simulink model "MainAssembly1"  (R2023a)
settings: Solver=VariableStepAuto  StartTime=0.0  StopTime=0.25  RelTol=1e-3
model workspace: external: MATLAB File C:\Users\danen\Desktop\MQPTest\MainAssembly1_DataFile1.m (data not in the file)
values from neighbouring files (symbols this model uses):
  Ts = 1e-06    [MainAssembly1_DataFile1.m]
undefined symbols (not defined in the file or in its folder): DiscIntNeverNeededParam, smiData, X, Y, Z
libraries: sm_lib x165, fl_lib x20, nesl_utility x10, fl_ps_legacy_lib x8, spsUniversalBridgeLib x8, spsCurrentMeasurementLib x8, spsDCVoltageSourceLib x4, spsStepperMotorLib x4, ee_lib x2, simulink x1, sps_lib x1
(part 1 of 4)
settings Model: Creator=danen  LastModifiedBy=danen

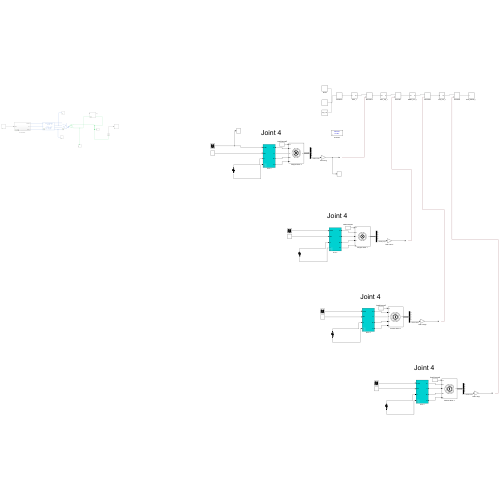
[thumbnail: Simulink's stored preview of the top-level diagram]
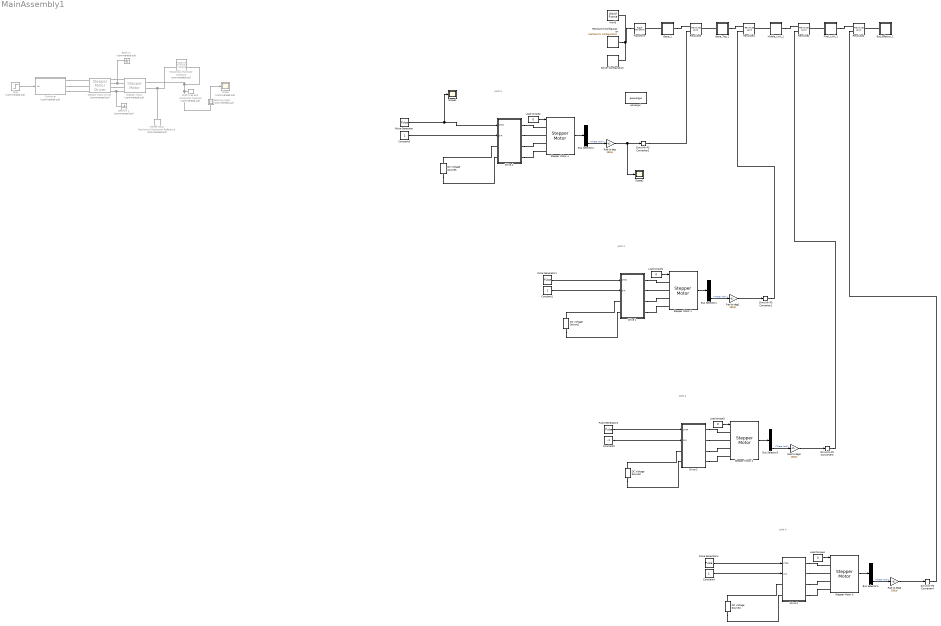
== system MainAssembly1 ==
  note: Joint 4
  note: Joint 4
  note: Joint 4
  note: Joint 4
  Base_1 : Subsystem
  Base_Top_1 : Subsystem
  Bus Selector{1..4} (4 alike) : BusSelector  OutputSignals=Vph (V),Iph (A),Te (N*m),w (rad/s),Theta (rad)
  Constant1 : Constant
  Constant2 : Constant  Value=-1
  Constant3 : Constant
  Constant4 : Constant
  Controller : Subsystem  Commented=on  Variant=on  VariantControlMode=label  LabelModeActiveChoice=Position
      settings: AttributesFormatString=%<BlockChoice>
  DC Voltage Source{1..4} (4 alike) : spsDCVoltageSourceLib/DC Voltage Source  Amplitude=5  Measurements=None
  Drive 1 : Subsystem  mask{Iref=2, step=500, Ts=Ts}
      mask prompts: Iref "Phase current (A)"; step "Stepping rate (step/s)"; Ts "Sampling time (s)"
      mask init:
      | Nstep=round(1/step/Ts);
  Drive 2 : Subsystem  mask{Iref=2, step=500, Ts=Ts}
      mask prompts: Iref "Phase current (A)"; step "Stepping rate (step/s)"; Ts "Sampling time (s)"
      mask init:
      | Nstep=round(1/step/Ts);
  Drive 3 : Subsystem  mask{Iref=2, step=500, Ts=Ts}
      mask prompts: Iref "Phase current (A)"; step "Stepping rate (step/s)"; Ts "Sampling time (s)"
      mask init:
      | Nstep=round(1/step/Ts);
  Drive 4 : Subsystem  mask{Iref=2, step=500, Ts=Ts}
      mask prompts: Iref "Phase current (A)"; step "Stepping rate (step/s)"; Ts "Sampling time (s)"
      mask init:
      | Nstep=round(1/step/Ts);
  ERef A+ : fl_lib/Electrical/Electrical Elements/Electrical Reference  Commented=on
  ERef A+1 : fl_lib/Electrical/Electrical Elements/Electrical Reference  Commented=on
  End_Effector_1 : Subsystem
  Final_Link_1 : Subsystem
  Load torque{1..4} (4 alike) : Constant  Value=0
  MRRef Motor : fl_lib/Mechanical/Rotational Elements/Mechanical Rotational Reference  Commented=on
  MechanismConfiguration : sm_lib/Utilities/Mechanism Configuration  UniformGravity=Constant  GravityVector=[0 -9.80665 0]  GravityVectorUnits=m/s^2  LinearizationDelta=0.001  JointModeTransitionNonlinearIterations=2
  Middle_Link_1 : Subsystem
  Pulse Generator : DiscretePulseGenerator  PulseType=Time based  Period=0.2  PulseWidth=0.5
  Pulse Generator1 : DiscretePulseGenerator  PulseType=Time based  Period=0.1  PulseWidth=0.1
  Pulse Generator2 : DiscretePulseGenerator  PulseType=Time based  Period=0.1  PulseWidth=0.1
  Pulse Generator4 : DiscretePulseGenerator  PulseType=Time based  Period=0.1  PulseWidth=0.1
  Rad to deg{,1..3} (4 alike) : Gain  Gain=180/pi
  Revolute1 : sm_lib/Joints/Revolute Joint  JointMode=Normal  SenseConstraintForce=off  SenseConstraintForceX=off  SenseConstraintForceY=off  SenseConstraintForceZ=off  SenseConstraintTorque=off  SenseConstraintTorqueX=off  SenseConstraintTorqueY=off  SenseConstraintTorqueZ=off  SenseTotalForce=off  SenseTotalForceX=off  SenseTotalForceY=off  SenseTotalForceZ=off  SenseTotalTorque=off  SenseTotalTorqueX=off  SenseTotalTorqueY=off  SenseTotalTorqueZ=off  CompositeWrenchDir=FollowerOnBase  CompositeWrenchFrame=BaseFrame  EquilibriumPosition=0  EquilibriumPositionUnits=deg  SpringStiffness=0  SpringStiffnessUnits=N*m/deg  DampingCoefficient=0  DampingCoefficientUnits=N*m/(deg/s)  TorqueActuationMode=ComputedTorque  MotionActuationMode=InputMotion  SensePosition=off  SenseVelocity=off  SenseAcceleration=off  SenseTorqueForce=off  SenseLowerLimitTorqueForce=off  SenseUpperLimitTorqueForce=off  LowerLimitSpecify=off  LowerLimitBound=-90  LowerLimitBoundUnits=deg  LowerLimitStiffness=1e4  LowerLimitStiffnessUnits=N*m/deg  LowerLimitDamping=10  LowerLimitDampingUnits=N*m/(deg/s)  LowerLimitTransitionRegionWidth=0.1  LowerLimitTransitionRegionWidthUnits=deg  UpperLimitSpecify=off  UpperLimitBound=90  UpperLimitBoundUnits=deg  UpperLimitStiffness=1e4  UpperLimitStiffnessUnits=N*m/deg  UpperLimitDamping=10  UpperLimitDampingUnits=N*m/(deg/s)  UpperLimitTransitionRegionWidth=0.1  UpperLimitTransitionRegionWidthUnits=deg  PositionTargetSpecify=on  PositionTargetPriority=Low  PositionTargetValue=smiData.RevoluteJoint(3).Rz.Pos  PositionTargetValueUnits=deg  VelocityTargetSpecify=off  VelocityTargetPriority=High  VelocityTargetValue=0  VelocityTargetValueUnits=deg/s
  Revolute2 : sm_lib/Joints/Revolute Joint  JointMode=Normal  SenseConstraintForce=off  SenseConstraintForceX=off  SenseConstraintForceY=off  SenseConstraintForceZ=off  SenseConstraintTorque=off  SenseConstraintTorqueX=off  SenseConstraintTorqueY=off  SenseConstraintTorqueZ=off  SenseTotalForce=off  SenseTotalForceX=off  SenseTotalForceY=off  SenseTotalForceZ=off  SenseTotalTorque=off  SenseTotalTorqueX=off  SenseTotalTorqueY=off  SenseTotalTorqueZ=off  CompositeWrenchDir=FollowerOnBase  CompositeWrenchFrame=BaseFrame  EquilibriumPosition=0  EquilibriumPositionUnits=deg  SpringStiffness=0  SpringStiffnessUnits=N*m/deg  DampingCoefficient=0  DampingCoefficientUnits=N*m/(deg/s)  TorqueActuationMode=ComputedTorque  MotionActuationMode=InputMotion  SensePosition=off  SenseVelocity=off  SenseAcceleration=off  SenseTorqueForce=off  SenseLowerLimitTorqueForce=off  SenseUpperLimitTorqueForce=off  LowerLimitSpecify=off  LowerLimitBound=-90  LowerLimitBoundUnits=deg  LowerLimitStiffness=1e4  LowerLimitStiffnessUnits=N*m/deg  LowerLimitDamping=10  LowerLimitDampingUnits=N*m/(deg/s)  LowerLimitTransitionRegionWidth=0.1  LowerLimitTransitionRegionWidthUnits=deg  UpperLimitSpecify=off  UpperLimitBound=90  UpperLimitBoundUnits=deg  UpperLimitStiffness=1e4  UpperLimitStiffnessUnits=N*m/deg  UpperLimitDamping=10  UpperLimitDampingUnits=N*m/(deg/s)  UpperLimitTransitionRegionWidth=0.1  UpperLimitTransitionRegionWidthUnits=deg  PositionTargetSpecify=on  PositionTargetPriority=Low  PositionTargetValue=smiData.RevoluteJoint(1).Rz.Pos  PositionTargetValueUnits=deg  VelocityTargetSpecify=off  VelocityTargetPriority=High  VelocityTargetValue=0  VelocityTargetValueUnits=deg/s
  Revolute3 : sm_lib/Joints/Revolute Joint  JointMode=Normal  SenseConstraintForce=off  SenseConstraintForceX=off  SenseConstraintForceY=off  SenseConstraintForceZ=off  SenseConstraintTorque=off  SenseConstraintTorqueX=off  SenseConstraintTorqueY=off  SenseConstraintTorqueZ=off  SenseTotalForce=off  SenseTotalForceX=off  SenseTotalForceY=off  SenseTotalForceZ=off  SenseTotalTorque=off  SenseTotalTorqueX=off  SenseTotalTorqueY=off  SenseTotalTorqueZ=off  CompositeWrenchDir=FollowerOnBase  CompositeWrenchFrame=BaseFrame  EquilibriumPosition=0  EquilibriumPositionUnits=deg  SpringStiffness=0  SpringStiffnessUnits=N*m/deg  DampingCoefficient=0  DampingCoefficientUnits=N*m/(deg/s)  TorqueActuationMode=ComputedTorque  MotionActuationMode=InputMotion  SensePosition=off  SenseVelocity=off  SenseAcceleration=off  SenseTorqueForce=off  SenseLowerLimitTorqueForce=off  SenseUpperLimitTorqueForce=off  LowerLimitSpecify=off  LowerLimitBound=-90  LowerLimitBoundUnits=deg  LowerLimitStiffness=1e4  LowerLimitStiffnessUnits=N*m/deg  LowerLimitDamping=10  LowerLimitDampingUnits=N*m/(deg/s)  LowerLimitTransitionRegionWidth=0.1  LowerLimitTransitionRegionWidthUnits=deg  UpperLimitSpecify=off  UpperLimitBound=90  UpperLimitBoundUnits=deg  UpperLimitStiffness=1e4  UpperLimitStiffnessUnits=N*m/deg  UpperLimitDamping=10  UpperLimitDampingUnits=N*m/(deg/s)  UpperLimitTransitionRegionWidth=0.1  UpperLimitTransitionRegionWidthUnits=deg  PositionTargetSpecify=on  PositionTargetPriority=Low  PositionTargetValue=smiData.RevoluteJoint(4).Rz.Pos  PositionTargetValueUnits=deg  VelocityTargetSpecify=off  VelocityTargetPriority=High  VelocityTargetValue=0  VelocityTargetValueUnits=deg/s
  Revolute4 : sm_lib/Joints/Revolute Joint  JointMode=Normal  SenseConstraintForce=off  SenseConstraintForceX=off  SenseConstraintForceY=off  SenseConstraintForceZ=off  SenseConstraintTorque=off  SenseConstraintTorqueX=off  SenseConstraintTorqueY=off  SenseConstraintTorqueZ=off  SenseTotalForce=off  SenseTotalForceX=off  SenseTotalForceY=off  SenseTotalForceZ=off  SenseTotalTorque=off  SenseTotalTorqueX=off  SenseTotalTorqueY=off  SenseTotalTorqueZ=off  CompositeWrenchDir=FollowerOnBase  CompositeWrenchFrame=BaseFrame  EquilibriumPosition=0  EquilibriumPositionUnits=deg  SpringStiffness=0  SpringStiffnessUnits=N*m/deg  DampingCoefficient=0  DampingCoefficientUnits=N*m/(deg/s)  TorqueActuationMode=ComputedTorque  MotionActuationMode=InputMotion  SensePosition=off  SenseVelocity=off  SenseAcceleration=off  SenseTorqueForce=off  SenseLowerLimitTorqueForce=off  SenseUpperLimitTorqueForce=off  LowerLimitSpecify=off  LowerLimitBound=-90  LowerLimitBoundUnits=deg  LowerLimitStiffness=1e4  LowerLimitStiffnessUnits=N*m/deg  LowerLimitDamping=10  LowerLimitDampingUnits=N*m/(deg/s)  LowerLimitTransitionRegionWidth=0.1  LowerLimitTransitionRegionWidthUnits=deg  UpperLimitSpecify=off  UpperLimitBound=90  UpperLimitBoundUnits=deg  UpperLimitStiffness=1e4  UpperLimitStiffnessUnits=N*m/deg  UpperLimitDamping=10  UpperLimitDampingUnits=N*m/(deg/s)  UpperLimitTransitionRegionWidth=0.1  UpperLimitTransitionRegionWidthUnits=deg  PositionTargetSpecify=on  PositionTargetPriority=Low  PositionTargetValue=smiData.RevoluteJoint(2).Rz.Pos  PositionTargetValueUnits=deg  VelocityTargetSpecify=off  VelocityTargetPriority=High  VelocityTargetValue=0  VelocityTargetValueUnits=deg/s
  Rotational Multibody Interface : fl_lib/Mechanical/Multibody Interfaces/Rotational Multibody Interface  Commented=on
  Scope : Scope  Commented=on
  Scope1 : Scope
  Scope2 : Scope
  Sensing Angle : Subsystem  Commented=on
      mask Display: disp('a')
  Shaft Free End : fl_lib/Mechanical/Rotational Elements/Rotational Free End  Commented=on  w_specify=off  w_priority=None  w=0 rad/s  w_nominal_specify=off  w_nominal_unit=rad/s  w_nominal_value=1
  Simulink-PS Converter{1..4} (4 alike) : nesl_utility/Simulink-PS Converter  PhysicalDomain=network_engine_domain  SubClassName=ps_input  LeftPortType=input  RightPortType=output  PseudoPeriodic=off  Frequencies=[]  NoiseDistribution=none  NoiseParameters=[]  Unit=1  AffineConversion=off  FilteringAndDerivatives=zero  SimscapeFilterOrder=1  InputFilterTimeConstant=0.001  UdotUserProvided=0
  Solver Configuration : nesl_utility/Solver Configuration  PhysicalDomain=network_engine_domain  SubClassName=solver  LeftPortType=input  RightPortType=generic  Tones=[]  Harmonics=[]  SimulateNoise=off  Profile=off  UseLocalSampling=off  EnableSwitchedLinearOptims=on  FrequencyDomain=off  UseCCode=off  RelTol=0.001  AbsTol=0.001  MinStep=1e-09  ToWorkspace=off  RevertToSquareIcSolve=off  NumHomotopyIterations=100  PhasorMode=off  PhasorModeNumHarmonics=1  ConsistencySolver=NEWTON_XTOL_AFTER_FTOL  IndexReductionMethod=DerivativeReplacement  DoDC=off  ResidualTolerance=1e-09  ConsistencyTolSource=GLOBAL  ConsistencyAbsTol=0.001  ConsistencyRelTol=0.001  ConsistencyTolFactor=0.001  UseLocalSolver=off  LocalSolverChoice=NE_BACKWARD_EULER_ADVANCER  ResolveIndetEquations=on  FunctionEvalNumThread=1  LocalSolverSampleTime=0.001  DoFixedCost=off  MaxNonlinIter=3  MaxModeIter=2  ComputeImpulses=off  ImpulseIterations=2  LinearAlgebra=auto  LinearAlgebraNumThread=0  EquationFormulation=NE_TIME_EF  DelaysMemoryBudget=1024  AutomaticFiltering=on  FilteringTimeConstant=0.001  PartitionStorageMethod=AS_NEEDED  PartitionMemoryBudget=1024  PartitionMethod=ROBUST
  Step : Step  Commented=on  Before=50  After=0  SampleTime=0
  Stepper Motor : ee_lib/Electromechanical/Reluctance & Stepper/Stepper Motor  Commented=on  step_or_av=ee.enum.electromech.simulationMode.stepping  Ra=0.55 Ohm  La=1.5e-3 H  Km=0.19 N*m/A  Td=0 N*m  Rm=inf Ohm  w_vec=[0, 1000, 3000] rpm  T_vec=[2, 2, 1] N*m  assert_if_slipping=ee.enum.assertAction.none  J_total=1e-4 kg*m^2  max_step_rate=10 Hz  Step=1.8 deg  J=4.5e-5 kg*m^2  B=8.0e-4 N*m*s/rad  speed0=0 rpm  theta0=0 deg  alpha=[.00393, .00393] 1/K  Tmeas=25 degC  Tmeas2=125 degC  T_vec2=[1.7, 1.7, .85] N*m  half_stepping=ee.enum.electromech.steppingModeAveraged.fullStep  thermal_masses=[100, 100] J/K  initial_temperatures=[25, 25] degC  rotor_thermal_mass=50 J/K  rotor_initial_temperature=25 degC  Rm_percent_rotor=90
      settings: InternalSimscapePortConfiguration="{\"Bottom\":[],\"Left\":[{\"id\":\"pA\",\"label\":\"A+\",\"type\":\"foundation.electrical.electrical\"},{\"id\":\"nA\",\"label\":\"A-\",\"type\":\"foundation.electrical.electrical\"},{\"id\":\"pB\",\"label\":\"B+\",\"type\":\"foundation.electrical.electrical\"},{\"id\":\"nB\",\"label\":\"B-\",\"type\":\"foundation.electrical.electrical\"}],\"Right\":[{\"id\":\"R\",\"label\":\"R\",\"type\":\"foundation.mechanical.rotational.rotational\"},{\"id\":\"C\",\"label\":\"C\",\"type\":\"foundation.mechanical.rotational.rotational\"}],\"Top\":[]}"
  Stepper Motor 1 : spsStepperMotorLib/Stepper Motor  MotorType=Permanent-magnet / Hybrid  NumberOfPhases_1=2  NumberOfPhases_2=3  PresetModel_1=<empty>  PresetModel_2=<empty>  L=3e-3  Lmax=10e-3  Lmin=2e-3  R=1.4  Step_angle=1.8  Psim=0.04  Tdm=0.02  J=1e-4/5  B=1e-3  w0=0  pos0=0  TsPowergui=0  TsBlock=-1
      settings: LibrarySourceBlock=sps_lib/Electrical Machines/Stepper Motor
  Stepper Motor 2 : spsStepperMotorLib/Stepper Motor  MotorType=Permanent-magnet / Hybrid  NumberOfPhases_1=2  NumberOfPhases_2=3  PresetModel_1=<empty>  PresetModel_2=<empty>  L=3e-3  Lmax=10e-3  Lmin=2e-3  R=1.4  Step_angle=1.8  Psim=0.04  Tdm=0.02  J=1e-4/5  B=1e-3  w0=0  pos0=0  TsPowergui=0  TsBlock=-1
      settings: LibrarySourceBlock=sps_lib/Electrical Machines/Stepper Motor
  Stepper Motor 3 : spsStepperMotorLib/Stepper Motor  MotorType=Permanent-magnet / Hybrid  NumberOfPhases_1=2  NumberOfPhases_2=3  PresetModel_1=<empty>  PresetModel_2=<empty>  L=3e-3  Lmax=10e-3  Lmin=2e-3  R=1.4  Step_angle=1.8  Psim=0.04  Tdm=0.02  J=1e-4/5  B=1e-3  w0=0  pos0=0  TsPowergui=0  TsBlock=-1
      settings: LibrarySourceBlock=sps_lib/Electrical Machines/Stepper Motor
  Stepper Motor 4 : spsStepperMotorLib/Stepper Motor  MotorType=Permanent-magnet / Hybrid  NumberOfPhases_1=2  NumberOfPhases_2=3  PresetModel_1=<empty>  PresetModel_2=<empty>  L=3e-3  Lmax=10e-3  Lmin=2e-3  R=1.4  Step_angle=1.8  Psim=0.04  Tdm=0.02  J=1e-4/5  B=1e-3  w0=0  pos0=180  TsPowergui=0  TsBlock=-1
      settings: LibrarySourceBlock=sps_lib/Electrical Machines/Stepper Motor
  Stepper Motor Driver : ee_lib/Electromechanical/Reluctance & Stepper/Stepper Motor Driver  Commented=on  step_or_av=ee.enum.electromech.simulationMode.stepping  step_rate_per_volt=10 Hz/V  Venable=2.5 V  Vreverse=2.5 V  supply_ports=ee.enum.supply_ports.hidesupply  Vm=5 V  Vsupply=10 V  half_stepping=ee.enum.electromech.steppingModeAveraged.fullStep  stepping_mode=ee.enum.electromech.steppingMode.fullStep  numMicroSteps=4  Im=1.2 A
      settings: InternalSimscapePortConfiguration="{\"Bottom\":[],\"Left\":[{\"id\":\"ENA\",\"label\":\"ENA\",\"type\":\"foundation.electrical.electrical\"},{\"id\":\"REF\",\"label\":\"REF\",\"type\":\"foundation.electrical.electrical\"},{\"id\":\"REV\",\"label\":\"REV\",\"type\":\"foundation.electrical.electrical\"}],\"Right\":[{\"id\":\"pA\",\"label\":\"A+\",\"type\":\"foundation.electrical.electrical\"},{\"id\":\"nA\",\"label\":\"A-\",\"type\":\"foundation.electrical.electrical\"},{\"id\":\"pB\",\"label\":\"B+\",\"type\":\"foundation.electrical.electrical\"},{\"id\":\"nB\",\"label\":\"B-\",\"type\":\"foundation.electrical.electrical\"}],\"Top\":[]}"
  Transform : sm_lib/Frames and Transforms/Rigid Transform  TranslationMethod=Cartesian  TranslationStandardOffset=0  TranslationStandardOffsetUnits=m  TranslationStandardAxis=+Z  TranslationCartesianOffset=smiData.RigidTransform(66).translation  TranslationCartesianOffsetUnits=m  TranslationROffset=0  TranslationROffsetUnits=m  TranslationZOffset=0  TranslationZOffsetUnits=m  TranslationThetaOffset=0  TranslationThetaOffsetUnits=deg  RotationMethod=ArbitraryAxis  RotationAngleUnits=rad  RotationStandardAxis=+Z  RotationAngle=smiData.RigidTransform(66).angle  RotationArbitraryAxis=smiData.RigidTransform(66).axis  FollAlignAxisA=+X  BaseAlignAxisA=+Y  FollAlignAxisB=+Y  BaseAlignAxisB=+Z  RotationSequenceAxes=FollowerAxes  RotationSequence=XYX  RotationSequenceAngles=[0 0 0]  RotationSequenceAnglesUnits=deg  RotationMatrix=[1 0 0; 0 1 0; 0 0 1]  Quaternion=[1 0 0 0]
  World : sm_lib/Frames and Transforms/World Frame
  powergui : sps_lib/powergui  Priority=1  SimulationMode=Discrete  SampleTime=Ts  frequency=60  Iterations=50  frequencyindice=0  Pbase=100e6  ErrMax=1e-4  UnitsV=kV  UnitsW=MW  buscounter=0  FunctionMessages=off  echomessages=off  EnableUseOfTLC=off  CurrentSourceSwitches=off  DisableSnubberDevices=off  DisableRonSwitches=off  DisableVfSwitches=off  DisplayEquations=off  AutomaticDiscreteSolvers=off  SolverType=Tustin/Backward Euler (TBE)  Interpol=off  ExternalGateDelay=off  methode=off  Ts=100  x0status=blocks  SPID=on  SwTol=0  HookPort=off  NonlinearTolerance=1e-4  nMaxIteration=100  ContinueOnMaxIteration=off  RestoreLinks=warning  ResistiveCurrentMeasurement=off  Frange=[0:2:500]  Ylog=off  Xlog=on  ShowGrid=off  save=off  variable=ZData  structure=0  ZoomFFT=off  StartTime=0.0  cycles=1  DisplayStyle=1  fundamental=60  FreqAxis=off  MaxFrequency=1000  frequencyindicesteady=1  RmsSteady=1  display=off
  wires:
  Rad to deg/1 -> Scope2/1, Simulink-PS Converter2/1
  Constant3/1 -> Drive 4/2(DIR)
  Pulse Generator/1 -> Scope1/1, Drive 4/1(STEP)
  Stepper Motor 4/1 -> Bus Selector2/1
  Bus Selector2/5 -> Rad to deg/1  "<Theta (rad)>"
  Load torque2/1 -> Stepper Motor 4/1
  Step/1 -> Controller/1(Ref)
  Sensing Angle/1(theta) -> Scope/1
  Bus Selector1/5 -> Rad to deg1/1  "<Theta (rad)>"
  Constant1/1 -> Drive 1/2(DIR)
  Stepper Motor 1/1 -> Bus Selector1/1
  Rad to deg1/1 -> Simulink-PS Converter1/1
  Load torque1/1 -> Stepper Motor 1/1
  Pulse Generator1/1 -> Drive 1/1(STEP)
  Bus Selector3/5 -> Rad to deg2/1  "<Theta (rad)>"
  Constant2/1 -> Drive 2/2(DIR)
  Stepper Motor 2/1 -> Bus Selector3/1
  Rad to deg2/1 -> Simulink-PS Converter3/1
  Load torque3/1 -> Stepper Motor 2/1
  Pulse Generator2/1 -> Drive 2/1(STEP)
  Bus Selector4/5 -> Rad to deg3/1  "<Theta (rad)>"
  Constant4/1 -> Drive 3/2(DIR)
  Stepper Motor 3/1 -> Bus Selector4/1
  Rad to deg3/1 -> Simulink-PS Converter4/1
  Load torque4/1 -> Stepper Motor 3/1
  Pulse Generator4/1 -> Drive 3/1(STEP)
  connections:
  Transform/LConn1 -- MechanismConfiguration/RConn1 -- Solver Configuration/RConn1 -- World/RConn1
  Base_1/LConn1 -- Transform/RConn1
  Middle_Link_1/RConn1 -- Revolute2/LConn1
  Final_Link_1/LConn1 -- Revolute2/RConn1
  Final_Link_1/RConn1 -- Revolute4/LConn1
  End_Effector_1/LConn1 -- Revolute4/RConn1
  Base_Top_1/RConn1 -- Revolute1/LConn1
  Middle_Link_1/LConn1 -- Revolute1/RConn1
  Base_1/RConn1 -- Revolute3/LConn1
  Base_Top_1/LConn1 -- Revolute3/RConn1
  DC Voltage Source3/RConn1 -- Drive 4/LConn1
  DC Voltage Source3/LConn1 -- Drive 4/LConn2
  Drive 4/RConn4 -- Stepper Motor 4/LConn4
  Drive 4/RConn3 -- Stepper Motor 4/LConn3
  Drive 4/RConn2 -- Stepper Motor 4/LConn2
  Drive 4/RConn1 -- Stepper Motor 4/LConn1
  Stepper Motor/RConn2 -- MRRef Motor/LConn1 -- Rotational Multibody Interface/LConn2
  Stepper Motor Driver/RConn1 -- Stepper Motor/LConn1
  Stepper Motor Driver/RConn2 -- ERef A+/LConn1 -- Stepper Motor/LConn2
  Stepper Motor Driver/RConn3 -- Stepper Motor/LConn3
  Stepper Motor Driver/RConn4 -- ERef A+1/LConn1 -- Stepper Motor/LConn4
  Controller/RConn1 -- Stepper Motor Driver/LConn1
  Controller/RConn2 -- Stepper Motor Driver/LConn2
  Controller/RConn3 -- Stepper Motor Driver/LConn3
  Stepper Motor/RConn1 -- Rotational Multibody Interface/RConn2 -- Shaft Free End/LConn1 -- Sensing Angle/LConn1
  DC Voltage Source1/LConn1 -- Drive 1/LConn2
  DC Voltage Source1/RConn1 -- Drive 1/LConn1
  Drive 1/RConn3 -- Stepper Motor 1/LConn3
  Drive 1/RConn1 -- Stepper Motor 1/LConn1
  Drive 1/RConn4 -- Stepper Motor 1/LConn4
  Drive 1/RConn2 -- Stepper Motor 1/LConn2
  DC Voltage Source2/LConn1 -- Drive 2/LConn2
  DC Voltage Source2/RConn1 -- Drive 2/LConn1
  Drive 2/RConn3 -- Stepper Motor 2/LConn3
  Drive 2/RConn1 -- Stepper Motor 2/LConn1
  Drive 2/RConn4 -- Stepper Motor 2/LConn4
  Drive 2/RConn2 -- Stepper Motor 2/LConn2
  DC Voltage Source4/LConn1 -- Drive 3/LConn2
  DC Voltage Source4/RConn1 -- Drive 3/LConn1
  Drive 3/RConn3 -- Stepper Motor 3/LConn3
  Drive 3/RConn1 -- Stepper Motor 3/LConn1
  Drive 3/RConn4 -- Stepper Motor 3/LConn4
  Drive 3/RConn2 -- Stepper Motor 3/LConn2
  Simulink-PS Converter2/RConn1 -- Revolute3/LConn2
  Simulink-PS Converter1/RConn1 -- Revolute1/LConn2
  Simulink-PS Converter3/RConn1 -- Revolute2/LConn2
  Simulink-PS Converter4/RConn1 -- Revolute4/LConn2

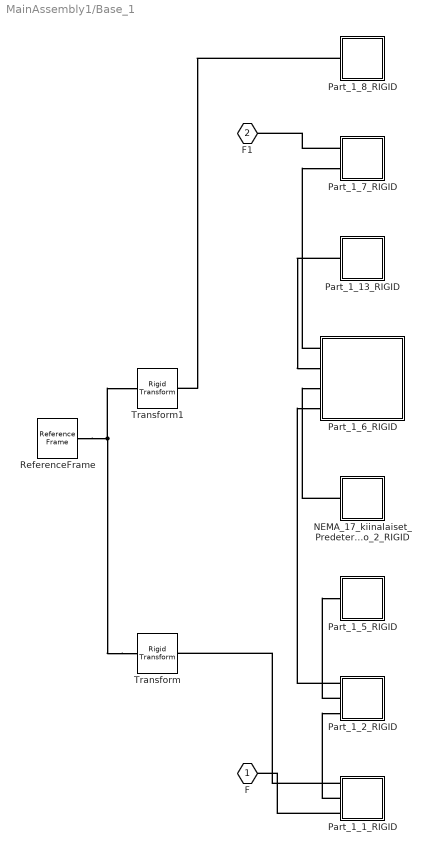
== system MainAssembly1/Base_1 ==
  NEMA_17_kiinalaiset_Predeterminado_2_RIGID : Subsystem
  Part_1_13_RIGID : Subsystem
  Part_1_1_RIGID : Subsystem
  Part_1_2_RIGID : Subsystem
  Part_1_5_RIGID : Subsystem
  Part_1_6_RIGID : Subsystem
  Part_1_7_RIGID : Subsystem
  Part_1_8_RIGID : Subsystem
  ReferenceFrame : sm_lib/Frames and Transforms/Reference Frame
  Transform : sm_lib/Frames and Transforms/Rigid Transform  TranslationMethod=Cartesian  TranslationStandardOffset=0  TranslationStandardOffsetUnits=m  TranslationStandardAxis=+Z  TranslationCartesianOffset=smiData.RigidTransform(41).translation  TranslationCartesianOffsetUnits=m  TranslationROffset=0  TranslationROffsetUnits=m  TranslationZOffset=0  TranslationZOffsetUnits=m  TranslationThetaOffset=0  TranslationThetaOffsetUnits=deg  RotationMethod=ArbitraryAxis  RotationAngleUnits=rad  RotationStandardAxis=+Z  RotationAngle=smiData.RigidTransform(41).angle  RotationArbitraryAxis=smiData.RigidTransform(41).axis  FollAlignAxisA=+X  BaseAlignAxisA=+Y  FollAlignAxisB=+Y  BaseAlignAxisB=+Z  RotationSequenceAxes=FollowerAxes  RotationSequence=XYX  RotationSequenceAngles=[0 0 0]  RotationSequenceAnglesUnits=deg  RotationMatrix=[1 0 0; 0 1 0; 0 0 1]  Quaternion=[1 0 0 0]
  Transform1 : sm_lib/Frames and Transforms/Rigid Transform  TranslationMethod=Cartesian  TranslationStandardOffset=0  TranslationStandardOffsetUnits=m  TranslationStandardAxis=+Z  TranslationCartesianOffset=smiData.RigidTransform(43).translation  TranslationCartesianOffsetUnits=m  TranslationROffset=0  TranslationROffsetUnits=m  TranslationZOffset=0  TranslationZOffsetUnits=m  TranslationThetaOffset=0  TranslationThetaOffsetUnits=deg  RotationMethod=ArbitraryAxis  RotationAngleUnits=rad  RotationStandardAxis=+Z  RotationAngle=smiData.RigidTransform(43).angle  RotationArbitraryAxis=smiData.RigidTransform(43).axis  FollAlignAxisA=+X  BaseAlignAxisA=+Y  FollAlignAxisB=+Y  BaseAlignAxisB=+Z  RotationSequenceAxes=FollowerAxes  RotationSequence=XYX  RotationSequenceAngles=[0 0 0]  RotationSequenceAnglesUnits=deg  RotationMatrix=[1 0 0; 0 1 0; 0 0 1]  Quaternion=[1 0 0 0]
  F : PMIOPort  Side=Left
  F1 : PMIOPort  Port=2  Side=Right
  connections:
  Transform/LConn1 -- ReferenceFrame/RConn1 -- Transform1/LConn1
  Part_1_1_RIGID/LConn1 -- Transform/RConn1
  Part_1_7_RIGID/LConn1 -- F1/RConn1
  Part_1_8_RIGID/LConn1 -- Transform1/RConn1
  Part_1_1_RIGID/LConn2 -- Part_1_2_RIGID/LConn3
  Part_1_2_RIGID/LConn1 -- Part_1_6_RIGID/LConn4
  Part_1_2_RIGID/LConn2 -- Part_1_5_RIGID/LConn1
  Part_1_13_RIGID/LConn1 -- Part_1_6_RIGID/LConn2
  NEMA_17_kiinalaiset_Predeterminado_2_RIGID/LConn1 -- Part_1_6_RIGID/LConn3
  Part_1_6_RIGID/LConn1 -- Part_1_7_RIGID/LConn2
  Part_1_1_RIGID/LConn3 -- F/RConn1

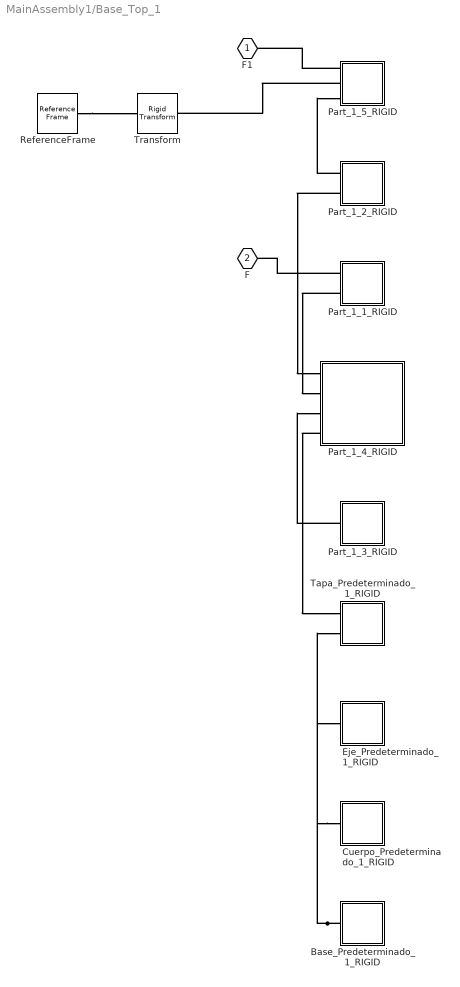
== system MainAssembly1/Base_Top_1 ==
  Base_Predeterminado_1_RIGID : Subsystem
  Cuerpo_Predeterminado_1_RIGID : Subsystem
  Eje_Predeterminado_1_RIGID : Subsystem
  Part_1_1_RIGID : Subsystem
  Part_1_2_RIGID : Subsystem
  Part_1_3_RIGID : Subsystem
  Part_1_4_RIGID : Subsystem
  Part_1_5_RIGID : Subsystem
  ReferenceFrame : sm_lib/Frames and Transforms/Reference Frame
  Tapa_Predeterminado_1_RIGID : Subsystem
  Transform : sm_lib/Frames and Transforms/Rigid Transform  TranslationMethod=Cartesian  TranslationStandardOffset=0  TranslationStandardOffsetUnits=m  TranslationStandardAxis=+Z  TranslationCartesianOffset=smiData.RigidTransform(24).translation  TranslationCartesianOffsetUnits=m  TranslationROffset=0  TranslationROffsetUnits=m  TranslationZOffset=0  TranslationZOffsetUnits=m  TranslationThetaOffset=0  TranslationThetaOffsetUnits=deg  RotationMethod=ArbitraryAxis  RotationAngleUnits=rad  RotationStandardAxis=+Z  RotationAngle=smiData.RigidTransform(24).angle  RotationArbitraryAxis=smiData.RigidTransform(24).axis  FollAlignAxisA=+X  BaseAlignAxisA=+Y  FollAlignAxisB=+Y  BaseAlignAxisB=+Z  RotationSequenceAxes=FollowerAxes  RotationSequence=XYX  RotationSequenceAngles=[0 0 0]  RotationSequenceAnglesUnits=deg  RotationMatrix=[1 0 0; 0 1 0; 0 0 1]  Quaternion=[1 0 0 0]
  F1 : PMIOPort  Side=Left
  F : PMIOPort  Port=2  Side=Right
  connections:
  Cuerpo_Predeterminado_1_RIGID/LConn1 -- Base_Predeterminado_1_RIGID/LConn1 -- Eje_Predeterminado_1_RIGID/LConn1 -- Tapa_Predeterminado_1_RIGID/LConn2
  ReferenceFrame/RConn1 -- Transform/LConn1
  Part_1_5_RIGID/LConn2 -- Transform/RConn1
  Part_1_3_RIGID/LConn1 -- Part_1_4_RIGID/LConn3
  Part_1_2_RIGID/LConn1 -- Part_1_5_RIGID/LConn3
  Part_1_2_RIGID/LConn2 -- Part_1_4_RIGID/LConn1
  Part_1_1_RIGID/LConn2 -- Part_1_4_RIGID/LConn2
  Part_1_4_RIGID/LConn4 -- Tapa_Predeterminado_1_RIGID/LConn1
  Part_1_1_RIGID/LConn1 -- F/RConn1
  Part_1_5_RIGID/LConn1 -- F1/RConn1

== system MainAssembly1/Controller ==
  Ref : Inport
  Position : Subsystem  VariantControl=Position
  Speed : Subsystem  VariantControl=Speed
  PWM : PMIOPort  Side=Right
  0v : PMIOPort  Port=2  Side=Right
  REV : PMIOPort  Port=3  Side=Right

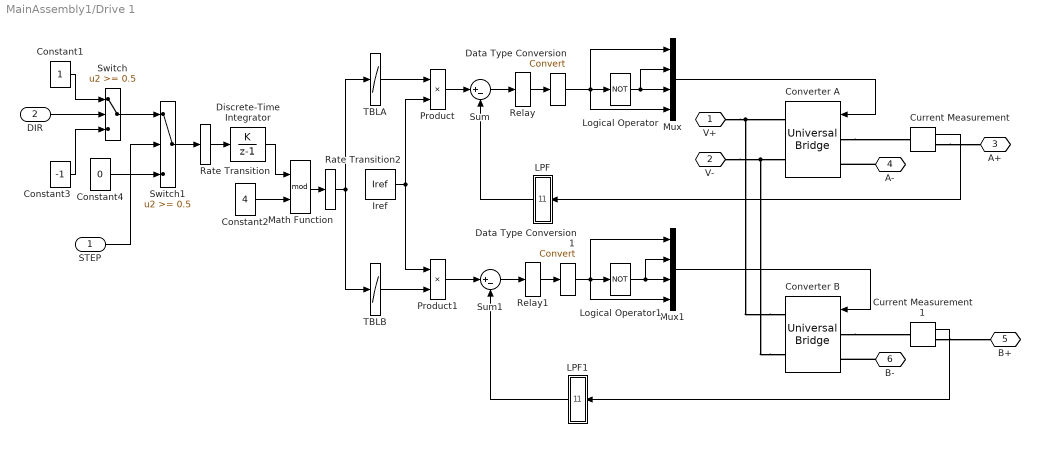
== system MainAssembly1/Drive 1 ==
  STEP : Inport
  DIR : Inport  Port=2
  Constant1 : Constant  SampleTime=Ts
  Constant2 : Constant  Value=4  SampleTime=Nstep*Ts
  Constant3 : Constant  Value=-1  SampleTime=Ts
  Constant4 : Constant  Value=0  SampleTime=Ts
  Converter A : spsUniversalBridgeLib/Universal Bridge  Arms=2  SnubberResistance=10000  SnubberCapacitance=inf  Device=MOSFET / Diodes  Ron=1e-3*10  Lon=0  ForwardVoltages="[  0  0  ]"  ForwardVoltage=0  GTOparameters=[ 10e-6 , 20e-6 ]  IGBTparameters=[ 0.5e-6 , 0.5e-6 ]  Measurements=None  Measurements_2=None  converterType=Rectifier
  Converter B : spsUniversalBridgeLib/Universal Bridge  Arms=2  SnubberResistance=10000  SnubberCapacitance=inf  Device=MOSFET / Diodes  Ron=1e-3*10  Lon=0  ForwardVoltages="[  0  0  ]"  ForwardVoltage=0  GTOparameters=[ 10e-6 , 20e-6 ]  IGBTparameters=[ 0.5e-6 , 0.5e-6 ]  Measurements=None  Measurements_2=None  converterType=Rectifier
  Current Measurement : spsCurrentMeasurementLib/Current Measurement  PhasorSimulation=off  OutputType=Complex  PSBequivalent=0
  Current Measurement1 : spsCurrentMeasurementLib/Current Measurement  PhasorSimulation=off  OutputType=Complex  PSBequivalent=0
  Data Type Conversion : DataTypeConversion  SaturateOnIntegerOverflow=off  RndMeth=Floor
  Data Type Conversion1 : DataTypeConversion  SaturateOnIntegerOverflow=off  RndMeth=Floor
  Discrete-Time Integrator : DiscreteIntegrator  IntegratorMethod=Accumulation: Forward Euler  SampleTime=Nstep*Ts  ICPrevOutput=DiscIntNeverNeededParam  ICPrevScaledInput=DiscIntNeverNeededParam
  Iref : Constant  Value=Iref  SampleTime=Ts
  LPF : Subsystem  mask{fc=10000, Ts=Ts}
      mask prompts: fc "Cut-off frequency (Hz)"; Ts "Sampling time (s)"
      mask init:
      | % fa=tf(1,[1/2/pi/fc 1]);
      | % fn=c2d(fa,Ts);
      | % [NN,DD]=tfdata(fn,'v')
      | 
      | NN = [ 0,0.0609];
      | DD = [1.0000,-0.9391];
  LPF1 : Subsystem  mask{fc=10000, Ts=Ts}
      mask prompts: fc "Cut-off frequency (Hz)"; Ts "Sampling time (s)"
      mask init:
      | % fa=tf(1,[1/2/pi/fc 1]);
      | % fn=c2d(fa,Ts);
      | % [NN,DD]=tfdata(fn,'v')
      | 
      | NN = [ 0,0.0609];
      | DD = [1.0000,-0.9391];
  Logical Operator : Logic  Operator=NOT  AllPortsSameDT=off  OutDataTypeStr=boolean
  Logical Operator1 : Logic  Operator=NOT  AllPortsSameDT=off  OutDataTypeStr=boolean
  Math Function : Math  Operator=mod  SignedPower=on  SampleTime=Nstep*Ts
  Mux : Mux
  Mux1 : Mux
  Product : Product  RndMeth=Zero
  Product1 : Product  RndMeth=Zero
  Rate Transition : RateTransition
  Rate Transition2 : RateTransition
  Relay : Relay  OnSwitchValue=0.01  OffSwitchValue=-0.01
  Relay1 : Relay  OnSwitchValue=0.01  OffSwitchValue=-0.01  OutDataTypeStr=Inherit: Inherit via back propagation
  Sum : Sum  Inputs=|+-  OutDataTypeStr=Inherit: Same as first input
  Sum1 : Sum  Inputs=|+-  OutDataTypeStr=Inherit: Same as first input
  Switch : Switch  Threshold=0.5  ZeroCross=off  SampleTime=Ts  SaturateOnIntegerOverflow=off  InputSameDT=off
  Switch1 : Switch  Threshold=0.5  ZeroCross=off  SampleTime=Ts  SaturateOnIntegerOverflow=off  InputSameDT=off
  TBLA : Lookup_n-D  NumberOfTableDimensions=1  BreakpointsForDimension1=[0:3]  BreakpointsForDimension2=[0 571.55 685.8 800.15 914.4 1028.8 1143.1 1257.4 1371.7 1486 1600.3 1714.6 1828.9 1943.2 2057.5 2171.8 2286.1 2400.5 2514.7 2629.1 2743.3 2857.7 2971.9 3086.3 3200.5 3314.9 3429.2]  Table=[1 0 -1 0]  InternalRulePriority=Speed  RndMeth=Simplest
  TBLB : Lookup_n-D  NumberOfTableDimensions=1  BreakpointsForDimension1=[0:3]  BreakpointsForDimension2=[0 571.55 685.8 800.15 914.4 1028.8 1143.1 1257.4 1371.7 1486 1600.3 1714.6 1828.9 1943.2 2057.5 2171.8 2286.1 2400.5 2514.7 2629.1 2743.3 2857.7 2971.9 3086.3 3200.5 3314.9 3429.2]  Table=[0 1 0 -1]  InternalRulePriority=Speed  RndMeth=Simplest
  V+ : PMIOPort  Side=Left
  V- : PMIOPort  Port=2  Side=Left
  A+ : PMIOPort  Port=3  Side=Right
  A- : PMIOPort  Port=4  Side=Right
  B+ : PMIOPort  Port=5  Side=Right
  B- : PMIOPort  Port=6  Side=Right
  wires:
  Constant4/1 -> Switch1/3
  Switch1/1 -> Rate Transition/1
  Switch/1 -> Switch1/1
  STEP/1 -> Switch1/2
  DIR/1 -> Switch/2
  Rate Transition2/1 -> TBLB/1, TBLA/1
  Math Function/1 -> Rate Transition2/1
  Product1/1 -> Sum1/1
  Product/1 -> Sum/1
  Rate Transition/1 -> Discrete-Time Integrator/1
  Constant3/1 -> Switch/3
  Constant1/1 -> Switch/1
  Discrete-Time Integrator/1 -> Math Function/1
  Constant2/1 -> Math Function/2
  Iref/1 -> Product1/1, Product/2
  TBLB/1 -> Product1/2
  TBLA/1 -> Product/1
  LPF1/1(O) -> Sum1/2
  LPF/1(O) -> Sum/2
  Data Type Conversion1/1 -> Mux1/4, Mux1/1, Logical Operator1/1
  Data Type Conversion/1 -> Logical Operator/1, Mux/4, Mux/1
  Current Measurement1/1 -> LPF1/1(I)
  Sum1/1 -> Relay1/1
  Mux1/1 -> Converter B/1
  Logical Operator1/1 -> Mux1/2, Mux1/3
  Relay1/1 -> Data Type Conversion1/1
  Mux/1 -> Converter A/1
  Logical Operator/1 -> Mux/2, Mux/3
  Relay/1 -> Data Type Conversion/1
  Current Measurement/1 -> LPF/1(I)
  Sum/1 -> Relay/1
  connections:
  Converter B/RConn2 -- Converter A/RConn2 -- V-/RConn1
  Converter B/RConn1 -- Converter A/RConn1 -- V+/RConn1
  Current Measurement1/RConn1 -- B+/RConn1
  Converter B/LConn1 -- Current Measurement1/LConn1
  Current Measurement/RConn1 -- A+/RConn1
  Converter A/LConn1 -- Current Measurement/LConn1
  B-/RConn1 -- Converter B/LConn2
  A-/RConn1 -- Converter A/LConn2

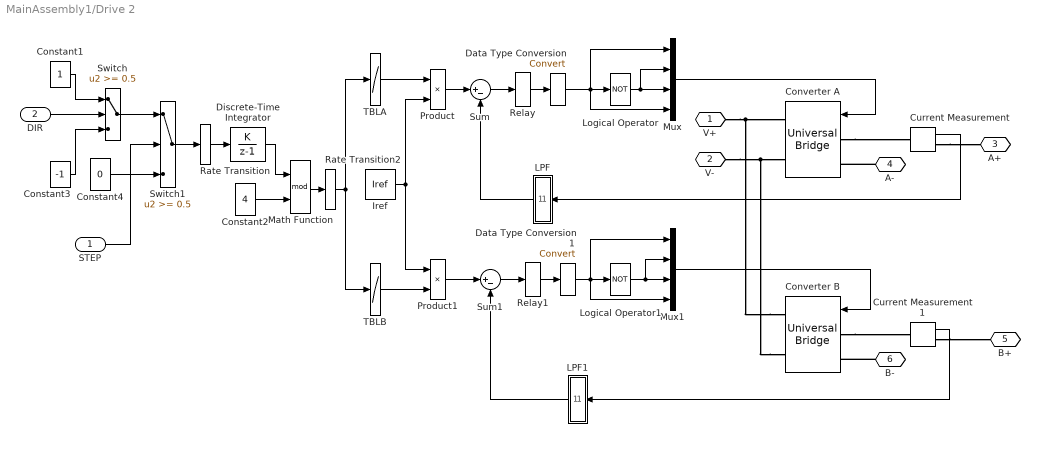
== system MainAssembly1/Drive 2 ==
  STEP : Inport
  DIR : Inport  Port=2
  Constant1 : Constant  SampleTime=Ts
  Constant2 : Constant  Value=4  SampleTime=Nstep*Ts
  Constant3 : Constant  Value=-1  SampleTime=Ts
  Constant4 : Constant  Value=0  SampleTime=Ts
  Converter A : spsUniversalBridgeLib/Universal Bridge  Arms=2  SnubberResistance=10000  SnubberCapacitance=inf  Device=MOSFET / Diodes  Ron=1e-3*10  Lon=0  ForwardVoltages="[  0  0  ]"  ForwardVoltage=0  GTOparameters=[ 10e-6 , 20e-6 ]  IGBTparameters=[ 0.5e-6 , 0.5e-6 ]  Measurements=None  Measurements_2=None  converterType=Rectifier
  Converter B : spsUniversalBridgeLib/Universal Bridge  Arms=2  SnubberResistance=10000  SnubberCapacitance=inf  Device=MOSFET / Diodes  Ron=1e-3*10  Lon=0  ForwardVoltages="[  0  0  ]"  ForwardVoltage=0  GTOparameters=[ 10e-6 , 20e-6 ]  IGBTparameters=[ 0.5e-6 , 0.5e-6 ]  Measurements=None  Measurements_2=None  converterType=Rectifier
  Current Measurement : spsCurrentMeasurementLib/Current Measurement  PhasorSimulation=off  OutputType=Complex  PSBequivalent=0
  Current Measurement1 : spsCurrentMeasurementLib/Current Measurement  PhasorSimulation=off  OutputType=Complex  PSBequivalent=0
  Data Type Conversion : DataTypeConversion  SaturateOnIntegerOverflow=off  RndMeth=Floor
  Data Type Conversion1 : DataTypeConversion  SaturateOnIntegerOverflow=off  RndMeth=Floor
  Discrete-Time Integrator : DiscreteIntegrator  IntegratorMethod=Accumulation: Forward Euler  SampleTime=Nstep*Ts  ICPrevOutput=DiscIntNeverNeededParam  ICPrevScaledInput=DiscIntNeverNeededParam
  Iref : Constant  Value=Iref  SampleTime=Ts
  LPF : Subsystem  mask{fc=10000, Ts=Ts}
      mask prompts: fc "Cut-off frequency (Hz)"; Ts "Sampling time (s)"
      mask init:
      | % fa=tf(1,[1/2/pi/fc 1]);
      | % fn=c2d(fa,Ts);
      | % [NN,DD]=tfdata(fn,'v')
      | 
      | NN = [ 0,0.0609];
      | DD = [1.0000,-0.9391];
  LPF1 : Subsystem  mask{fc=10000, Ts=Ts}
      mask prompts: fc "Cut-off frequency (Hz)"; Ts "Sampling time (s)"
      mask init:
      | % fa=tf(1,[1/2/pi/fc 1]);
      | % fn=c2d(fa,Ts);
      | % [NN,DD]=tfdata(fn,'v')
      | 
      | NN = [ 0,0.0609];
      | DD = [1.0000,-0.9391];
  Logical Operator : Logic  Operator=NOT  AllPortsSameDT=off  OutDataTypeStr=boolean
  Logical Operator1 : Logic  Operator=NOT  AllPortsSameDT=off  OutDataTypeStr=boolean
  Math Function : Math  Operator=mod  SignedPower=on  SampleTime=Nstep*Ts
  Mux : Mux
  Mux1 : Mux
  Product : Product  RndMeth=Zero
  Product1 : Product  RndMeth=Zero
  Rate Transition : RateTransition
  Rate Transition2 : RateTransition
  Relay : Relay  OnSwitchValue=0.01  OffSwitchValue=-0.01
  Relay1 : Relay  OnSwitchValue=0.01  OffSwitchValue=-0.01  OutDataTypeStr=Inherit: Inherit via back propagation
  Sum : Sum  Inputs=|+-  OutDataTypeStr=Inherit: Same as first input
  Sum1 : Sum  Inputs=|+-  OutDataTypeStr=Inherit: Same as first input
  Switch : Switch  Threshold=0.5  ZeroCross=off  SampleTime=Ts  SaturateOnIntegerOverflow=off  InputSameDT=off
  Switch1 : Switch  Threshold=0.5  ZeroCross=off  SampleTime=Ts  SaturateOnIntegerOverflow=off  InputSameDT=off
  TBLA : Lookup_n-D  NumberOfTableDimensions=1  BreakpointsForDimension1=[0:3]  BreakpointsForDimension2=[0 571.55 685.8 800.15 914.4 1028.8 1143.1 1257.4 1371.7 1486 1600.3 1714.6 1828.9 1943.2 2057.5 2171.8 2286.1 2400.5 2514.7 2629.1 2743.3 2857.7 2971.9 3086.3 3200.5 3314.9 3429.2]  Table=[1 0 -1 0]  InternalRulePriority=Speed  RndMeth=Simplest
  TBLB : Lookup_n-D  NumberOfTableDimensions=1  BreakpointsForDimension1=[0:3]  BreakpointsForDimension2=[0 571.55 685.8 800.15 914.4 1028.8 1143.1 1257.4 1371.7 1486 1600.3 1714.6 1828.9 1943.2 2057.5 2171.8 2286.1 2400.5 2514.7 2629.1 2743.3 2857.7 2971.9 3086.3 3200.5 3314.9 3429.2]  Table=[0 1 0 -1]  InternalRulePriority=Speed  RndMeth=Simplest
  V+ : PMIOPort  Side=Left
  V- : PMIOPort  Port=2  Side=Left
  A+ : PMIOPort  Port=3  Side=Right
  A- : PMIOPort  Port=4  Side=Right
  B+ : PMIOPort  Port=5  Side=Right
  B- : PMIOPort  Port=6  Side=Right
  wires:
  Constant4/1 -> Switch1/3
  Switch1/1 -> Rate Transition/1
  Switch/1 -> Switch1/1
  STEP/1 -> Switch1/2
  DIR/1 -> Switch/2
  Rate Transition2/1 -> TBLB/1, TBLA/1
  Math Function/1 -> Rate Transition2/1
  Product1/1 -> Sum1/1
  Product/1 -> Sum/1
  Rate Transition/1 -> Discrete-Time Integrator/1
  Constant3/1 -> Switch/3
  Constant1/1 -> Switch/1
  Discrete-Time Integrator/1 -> Math Function/1
  Constant2/1 -> Math Function/2
  Iref/1 -> Product1/1, Product/2
  TBLB/1 -> Product1/2
  TBLA/1 -> Product/1
  LPF1/1(O) -> Sum1/2
  LPF/1(O) -> Sum/2
  Data Type Conversion1/1 -> Mux1/4, Mux1/1, Logical Operator1/1
  Data Type Conversion/1 -> Logical Operator/1, Mux/4, Mux/1
  Current Measurement1/1 -> LPF1/1(I)
  Sum1/1 -> Relay1/1
  Mux1/1 -> Converter B/1
  Logical Operator1/1 -> Mux1/2, Mux1/3
  Relay1/1 -> Data Type Conversion1/1
  Mux/1 -> Converter A/1
  Logical Operator/1 -> Mux/2, Mux/3
  Relay/1 -> Data Type Conversion/1
  Current Measurement/1 -> LPF/1(I)
  Sum/1 -> Relay/1
  connections:
  Converter B/RConn2 -- Converter A/RConn2 -- V-/RConn1
  Converter B/RConn1 -- Converter A/RConn1 -- V+/RConn1
  Current Measurement1/RConn1 -- B+/RConn1
  Converter B/LConn1 -- Current Measurement1/LConn1
  Current Measurement/RConn1 -- A+/RConn1
  Converter A/LConn1 -- Current Measurement/LConn1
  B-/RConn1 -- Converter B/LConn2
  A-/RConn1 -- Converter A/LConn2

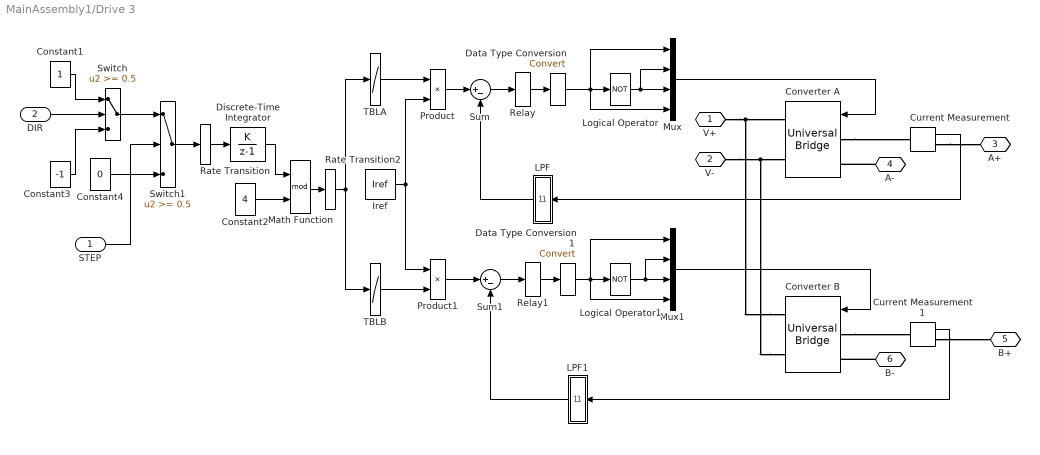
== system MainAssembly1/Drive 3 ==
  STEP : Inport
  DIR : Inport  Port=2
  Constant1 : Constant  SampleTime=Ts
  Constant2 : Constant  Value=4  SampleTime=Nstep*Ts
  Constant3 : Constant  Value=-1  SampleTime=Ts
  Constant4 : Constant  Value=0  SampleTime=Ts
  Converter A : spsUniversalBridgeLib/Universal Bridge  Arms=2  SnubberResistance=10000  SnubberCapacitance=inf  Device=MOSFET / Diodes  Ron=1e-3*10  Lon=0  ForwardVoltages="[  0  0  ]"  ForwardVoltage=0  GTOparameters=[ 10e-6 , 20e-6 ]  IGBTparameters=[ 0.5e-6 , 0.5e-6 ]  Measurements=None  Measurements_2=None  converterType=Rectifier
  Converter B : spsUniversalBridgeLib/Universal Bridge  Arms=2  SnubberResistance=10000  SnubberCapacitance=inf  Device=MOSFET / Diodes  Ron=1e-3*10  Lon=0  ForwardVoltages="[  0  0  ]"  ForwardVoltage=0  GTOparameters=[ 10e-6 , 20e-6 ]  IGBTparameters=[ 0.5e-6 , 0.5e-6 ]  Measurements=None  Measurements_2=None  converterType=Rectifier
  Current Measurement : spsCurrentMeasurementLib/Current Measurement  PhasorSimulation=off  OutputType=Complex  PSBequivalent=0
  Current Measurement1 : spsCurrentMeasurementLib/Current Measurement  PhasorSimulation=off  OutputType=Complex  PSBequivalent=0
  Data Type Conversion : DataTypeConversion  SaturateOnIntegerOverflow=off  RndMeth=Floor
  Data Type Conversion1 : DataTypeConversion  SaturateOnIntegerOverflow=off  RndMeth=Floor
  Discrete-Time Integrator : DiscreteIntegrator  IntegratorMethod=Accumulation: Forward Euler  SampleTime=Nstep*Ts  ICPrevOutput=DiscIntNeverNeededParam  ICPrevScaledInput=DiscIntNeverNeededParam
  Iref : Constant  Value=Iref  SampleTime=Ts
  LPF : Subsystem  mask{fc=10000, Ts=Ts}
      mask prompts: fc "Cut-off frequency (Hz)"; Ts "Sampling time (s)"
      mask init:
      | % fa=tf(1,[1/2/pi/fc 1]);
      | % fn=c2d(fa,Ts);
      | % [NN,DD]=tfdata(fn,'v')
      | 
      | NN = [ 0,0.0609];
      | DD = [1.0000,-0.9391];
  LPF1 : Subsystem  mask{fc=10000, Ts=Ts}
      mask prompts: fc "Cut-off frequency (Hz)"; Ts "Sampling time (s)"
      mask init:
      | % fa=tf(1,[1/2/pi/fc 1]);
      | % fn=c2d(fa,Ts);
      | % [NN,DD]=tfdata(fn,'v')
      | 
      | NN = [ 0,0.0609];
      | DD = [1.0000,-0.9391];
  Logical Operator : Logic  Operator=NOT  AllPortsSameDT=off  OutDataTypeStr=boolean
  Logical Operator1 : Logic  Operator=NOT  AllPortsSameDT=off  OutDataTypeStr=boolean
  Math Function : Math  Operator=mod  SignedPower=on  SampleTime=Nstep*Ts
  Mux : Mux
  Mux1 : Mux
  Product : Product  RndMeth=Zero
  Product1 : Product  RndMeth=Zero
  Rate Transition : RateTransition
  Rate Transition2 : RateTransition
  Relay : Relay  OnSwitchValue=0.01  OffSwitchValue=-0.01
  Relay1 : Relay  OnSwitchValue=0.01  OffSwitchValue=-0.01  OutDataTypeStr=Inherit: Inherit via back propagation
  Sum : Sum  Inputs=|+-  OutDataTypeStr=Inherit: Same as first input
  Sum1 : Sum  Inputs=|+-  OutDataTypeStr=Inherit: Same as first input
  Switch : Switch  Threshold=0.5  ZeroCross=off  SampleTime=Ts  SaturateOnIntegerOverflow=off  InputSameDT=off
  Switch1 : Switch  Threshold=0.5  ZeroCross=off  SampleTime=Ts  SaturateOnIntegerOverflow=off  InputSameDT=off
  TBLA : Lookup_n-D  NumberOfTableDimensions=1  BreakpointsForDimension1=[0:3]  BreakpointsForDimension2=[0 571.55 685.8 800.15 914.4 1028.8 1143.1 1257.4 1371.7 1486 1600.3 1714.6 1828.9 1943.2 2057.5 2171.8 2286.1 2400.5 2514.7 2629.1 2743.3 2857.7 2971.9 3086.3 3200.5 3314.9 3429.2]  Table=[1 0 -1 0]  InternalRulePriority=Speed  RndMeth=Simplest
  TBLB : Lookup_n-D  NumberOfTableDimensions=1  BreakpointsForDimension1=[0:3]  BreakpointsForDimension2=[0 571.55 685.8 800.15 914.4 1028.8 1143.1 1257.4 1371.7 1486 1600.3 1714.6 1828.9 1943.2 2057.5 2171.8 2286.1 2400.5 2514.7 2629.1 2743.3 2857.7 2971.9 3086.3 3200.5 3314.9 3429.2]  Table=[0 1 0 -1]  InternalRulePriority=Speed  RndMeth=Simplest
  V+ : PMIOPort  Side=Left
  V- : PMIOPort  Port=2  Side=Left
  A+ : PMIOPort  Port=3  Side=Right
  A- : PMIOPort  Port=4  Side=Right
  B+ : PMIOPort  Port=5  Side=Right
  B- : PMIOPort  Port=6  Side=Right
  wires:
  Constant4/1 -> Switch1/3
  Switch1/1 -> Rate Transition/1
  Switch/1 -> Switch1/1
  STEP/1 -> Switch1/2
  DIR/1 -> Switch/2
  Rate Transition2/1 -> TBLB/1, TBLA/1
  Math Function/1 -> Rate Transition2/1
  Product1/1 -> Sum1/1
  Product/1 -> Sum/1
  Rate Transition/1 -> Discrete-Time Integrator/1
  Constant3/1 -> Switch/3
  Constant1/1 -> Switch/1
  Discrete-Time Integrator/1 -> Math Function/1
  Constant2/1 -> Math Function/2
  Iref/1 -> Product1/1, Product/2
  TBLB/1 -> Product1/2
  TBLA/1 -> Product/1
  LPF1/1(O) -> Sum1/2
  LPF/1(O) -> Sum/2
  Data Type Conversion1/1 -> Mux1/4, Mux1/1, Logical Operator1/1
  Data Type Conversion/1 -> Logical Operator/1, Mux/4, Mux/1
  Current Measurement1/1 -> LPF1/1(I)
  Sum1/1 -> Relay1/1
  Mux1/1 -> Converter B/1
  Logical Operator1/1 -> Mux1/2, Mux1/3
  Relay1/1 -> Data Type Conversion1/1
  Mux/1 -> Converter A/1
  Logical Operator/1 -> Mux/2, Mux/3
  Relay/1 -> Data Type Conversion/1
  Current Measurement/1 -> LPF/1(I)
  Sum/1 -> Relay/1
  connections:
  Converter B/RConn2 -- Converter A/RConn2 -- V-/RConn1
  Converter B/RConn1 -- Converter A/RConn1 -- V+/RConn1
  Current Measurement1/RConn1 -- B+/RConn1
  Converter B/LConn1 -- Current Measurement1/LConn1
  Current Measurement/RConn1 -- A+/RConn1
  Converter A/LConn1 -- Current Measurement/LConn1
  B-/RConn1 -- Converter B/LConn2
  A-/RConn1 -- Converter A/LConn2

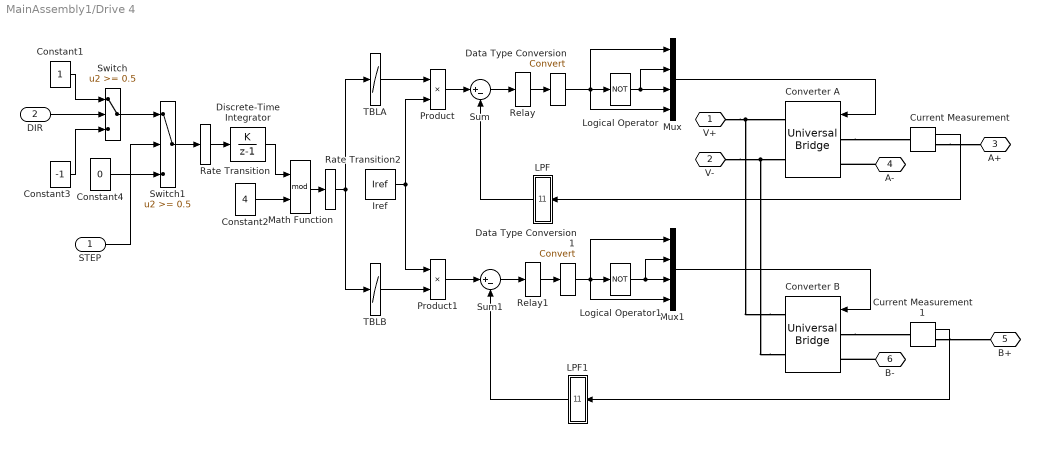
== system MainAssembly1/Drive 4 ==
  STEP : Inport
  DIR : Inport  Port=2
  Constant1 : Constant  SampleTime=Ts
  Constant2 : Constant  Value=4  SampleTime=Nstep*Ts
  Constant3 : Constant  Value=-1  SampleTime=Ts
  Constant4 : Constant  Value=0  SampleTime=Ts
  Converter A : spsUniversalBridgeLib/Universal Bridge  Arms=2  SnubberResistance=10000  SnubberCapacitance=inf  Device=MOSFET / Diodes  Ron=1e-3*10  Lon=0  ForwardVoltages="[  0  0  ]"  ForwardVoltage=0  GTOparameters=[ 10e-6 , 20e-6 ]  IGBTparameters=[ 0.5e-6 , 0.5e-6 ]  Measurements=None  Measurements_2=None  converterType=Rectifier
  Converter B : spsUniversalBridgeLib/Universal Bridge  Arms=2  SnubberResistance=10000  SnubberCapacitance=inf  Device=MOSFET / Diodes  Ron=1e-3*10  Lon=0  ForwardVoltages="[  0  0  ]"  ForwardVoltage=0  GTOparameters=[ 10e-6 , 20e-6 ]  IGBTparameters=[ 0.5e-6 , 0.5e-6 ]  Measurements=None  Measurements_2=None  converterType=Rectifier
  Current Measurement : spsCurrentMeasurementLib/Current Measurement  PhasorSimulation=off  OutputType=Complex  PSBequivalent=0
  Current Measurement1 : spsCurrentMeasurementLib/Current Measurement  PhasorSimulation=off  OutputType=Complex  PSBequivalent=0
  Data Type Conversion : DataTypeConversion  SaturateOnIntegerOverflow=off  RndMeth=Floor
  Data Type Conversion1 : DataTypeConversion  SaturateOnIntegerOverflow=off  RndMeth=Floor
  Discrete-Time Integrator : DiscreteIntegrator  IntegratorMethod=Accumulation: Forward Euler  SampleTime=Nstep*Ts  ICPrevOutput=DiscIntNeverNeededParam  ICPrevScaledInput=DiscIntNeverNeededParam
  Iref : Constant  Value=Iref  SampleTime=Ts
  LPF : Subsystem  mask{fc=10000, Ts=Ts}
      mask prompts: fc "Cut-off frequency (Hz)"; Ts "Sampling time (s)"
      mask init:
      | % fa=tf(1,[1/2/pi/fc 1]);
      | % fn=c2d(fa,Ts);
      | % [NN,DD]=tfdata(fn,'v')
      | 
      | NN = [ 0,0.0609];
      | DD = [1.0000,-0.9391];
  LPF1 : Subsystem  mask{fc=10000, Ts=Ts}
      mask prompts: fc "Cut-off frequency (Hz)"; Ts "Sampling time (s)"
      mask init:
      | % fa=tf(1,[1/2/pi/fc 1]);
      | % fn=c2d(fa,Ts);
      | % [NN,DD]=tfdata(fn,'v')
      | 
      | NN = [ 0,0.0609];
      | DD = [1.0000,-0.9391];
  Logical Operator : Logic  Operator=NOT  AllPortsSameDT=off  OutDataTypeStr=boolean
  Logical Operator1 : Logic  Operator=NOT  AllPortsSameDT=off  OutDataTypeStr=boolean
  Math Function : Math  Operator=mod  SignedPower=on  SampleTime=Nstep*Ts
  Mux : Mux
  Mux1 : Mux
  Product : Product  RndMeth=Zero
  Product1 : Product  RndMeth=Zero
  Rate Transition : RateTransition
  Rate Transition2 : RateTransition
  Relay : Relay  OnSwitchValue=0.01  OffSwitchValue=-0.01
  Relay1 : Relay  OnSwitchValue=0.01  OffSwitchValue=-0.01  OutDataTypeStr=Inherit: Inherit via back propagation
  Sum : Sum  Inputs=|+-  OutDataTypeStr=Inherit: Same as first input
  Sum1 : Sum  Inputs=|+-  OutDataTypeStr=Inherit: Same as first input
  Switch : Switch  Threshold=0.5  ZeroCross=off  SampleTime=Ts  SaturateOnIntegerOverflow=off  InputSameDT=off
  Switch1 : Switch  Threshold=0.5  ZeroCross=off  SampleTime=Ts  SaturateOnIntegerOverflow=off  InputSameDT=off
  TBLA : Lookup_n-D  NumberOfTableDimensions=1  BreakpointsForDimension1=[0:3]  BreakpointsForDimension2=[0 571.55 685.8 800.15 914.4 1028.8 1143.1 1257.4 1371.7 1486 1600.3 1714.6 1828.9 1943.2 2057.5 2171.8 2286.1 2400.5 2514.7 2629.1 2743.3 2857.7 2971.9 3086.3 3200.5 3314.9 3429.2]  Table=[1 0 -1 0]  InternalRulePriority=Speed  RndMeth=Simplest
  TBLB : Lookup_n-D  NumberOfTableDimensions=1  BreakpointsForDimension1=[0:3]  BreakpointsForDimension2=[0 571.55 685.8 800.15 914.4 1028.8 1143.1 1257.4 1371.7 1486 1600.3 1714.6 1828.9 1943.2 2057.5 2171.8 2286.1 2400.5 2514.7 2629.1 2743.3 2857.7 2971.9 3086.3 3200.5 3314.9 3429.2]  Table=[0 1 0 -1]  InternalRulePriority=Speed  RndMeth=Simplest
  V+ : PMIOPort  Side=Left
  V- : PMIOPort  Port=2  Side=Left
  A+ : PMIOPort  Port=3  Side=Right
  A- : PMIOPort  Port=4  Side=Right
  B+ : PMIOPort  Port=5  Side=Right
  B- : PMIOPort  Port=6  Side=Right
  wires:
  Constant4/1 -> Switch1/3
  Switch1/1 -> Rate Transition/1
  Switch/1 -> Switch1/1
  STEP/1 -> Switch1/2
  DIR/1 -> Switch/2
  Rate Transition2/1 -> TBLB/1, TBLA/1
  Math Function/1 -> Rate Transition2/1
  Product1/1 -> Sum1/1
  Product/1 -> Sum/1
  Rate Transition/1 -> Discrete-Time Integrator/1
  Constant3/1 -> Switch/3
  Constant1/1 -> Switch/1
  Discrete-Time Integrator/1 -> Math Function/1
  Constant2/1 -> Math Function/2
  Iref/1 -> Product1/1, Product/2
  TBLB/1 -> Product1/2
  TBLA/1 -> Product/1
  LPF1/1(O) -> Sum1/2
  LPF/1(O) -> Sum/2
  Data Type Conversion1/1 -> Mux1/4, Mux1/1, Logical Operator1/1
  Data Type Conversion/1 -> Logical Operator/1, Mux/4, Mux/1
  Current Measurement1/1 -> LPF1/1(I)
  Sum1/1 -> Relay1/1
  Mux1/1 -> Converter B/1
  Logical Operator1/1 -> Mux1/2, Mux1/3
  Relay1/1 -> Data Type Conversion1/1
  Mux/1 -> Converter A/1
  Logical Operator/1 -> Mux/2, Mux/3
  Relay/1 -> Data Type Conversion/1
  Current Measurement/1 -> LPF/1(I)
  Sum/1 -> Relay/1
  connections:
  Converter B/RConn2 -- Converter A/RConn2 -- V-/RConn1
  Converter B/RConn1 -- Converter A/RConn1 -- V+/RConn1
  Current Measurement1/RConn1 -- B+/RConn1
  Converter B/LConn1 -- Current Measurement1/LConn1
  Current Measurement/RConn1 -- A+/RConn1
  Converter A/LConn1 -- Current Measurement/LConn1
  B-/RConn1 -- Converter B/LConn2
  A-/RConn1 -- Converter A/LConn2

== system MainAssembly1/End_Effector_1 ==
  Claw_mount_copy_v1_1_RIGID : Subsystem
  Lazy_Susan_1_RIGID : Subsystem
  ReferenceFrame : sm_lib/Frames and Transforms/Reference Frame
  Transform : sm_lib/Frames and Transforms/Rigid Transform  TranslationMethod=Cartesian  TranslationStandardOffset=0  TranslationStandardOffsetUnits=m  TranslationStandardAxis=+Z  TranslationCartesianOffset=smiData.RigidTransform(36).translation  TranslationCartesianOffsetUnits=m  TranslationROffset=0  TranslationROffsetUnits=m  TranslationZOffset=0  TranslationZOffsetUnits=m  TranslationThetaOffset=0  TranslationThetaOffsetUnits=deg  RotationMethod=ArbitraryAxis  RotationAngleUnits=rad  RotationStandardAxis=+Z  RotationAngle=smiData.RigidTransform(36).angle  RotationArbitraryAxis=smiData.RigidTransform(36).axis  FollAlignAxisA=+X  BaseAlignAxisA=+Y  FollAlignAxisB=+Y  BaseAlignAxisB=+Z  RotationSequenceAxes=FollowerAxes  RotationSequence=XYX  RotationSequenceAngles=[0 0 0]  RotationSequenceAnglesUnits=deg  RotationMatrix=[1 0 0; 0 1 0; 0 0 1]  Quaternion=[1 0 0 0]
  x5mm_rod_1_RIGID : Subsystem
  F : PMIOPort  Side=Left
  connections:
  ReferenceFrame/RConn1 -- Transform/LConn1
  Lazy_Susan_1_RIGID/LConn3 -- Transform/RConn1
  Claw_mount_copy_v1_1_RIGID/LConn2 -- Lazy_Susan_1_RIGID/LConn1
  Claw_mount_copy_v1_1_RIGID/LConn1 -- x5mm_rod_1_RIGID/LConn1
  Lazy_Susan_1_RIGID/LConn2 -- F/RConn1
